simulink model "px4_rc_control"  (R2021b)
settings: Solver=FixedStepAuto  StartTime=0.0  StopTime=inf  RelTol=1e-3
undefined symbols (not defined in the file): A, B, G, R
libraries: robotlib x3, aerolibanimutils x1
settings Model: Creator=jawher  LastModifiedBy=jawher
settings OptimizationCC: EnhancedBackFolding=on  PassReuseOutputArgsAs=Individual arguments  ZeroExternalMemoryAtStartup=off  ZeroInternalMemoryAtStartup=off  MaxStackSize=64  OptimizeBlockOrder=speed  DifferentSizesBufferReuse=on  OptimizationCustomize=off  EfficientTunableParamExpr=on
settings DebuggingCC: ParameterTunabilityLossMsg=error
settings HardwareCC: ProdBitPerPointer=32  ProdBitPerSizeT=32  ProdBitPerPtrDiffT=32  ProdLargestAtomicFloat=None  ProdIntDivRoundTo=Undefined  ProdEndianess=Unspecified  ProdWordSize=32  ProdHWDeviceType=Generic->Unspecified (assume 32-bit Generic)
settings SFSimCC: MATLABDynamicMemAlloc=off
settings RTWCC: Description=Embedded Coder  SystemTargetFile=ert.tlc  HardwareBoard=Robot Operating System (ROS)  TLCOptions="-aInlineSetEventsForThisBaseRateFcn=TLC_FALSE -aSuppressMultiTaskScheduler=TLC_FALSE  -aRateBasedStepFcn=0"  TemplateMakefile=ert_default_tmf  Toolchain=Catkin  TargetLang=C++
settings CodeAppCC: ForceParamTrailComments=on  IgnoreCustomStorageClasses=off  OperatorAnnotations=on  SimulinkDataObjDesc=on  SFDataObjDesc=on  InsertBlockDesc=on

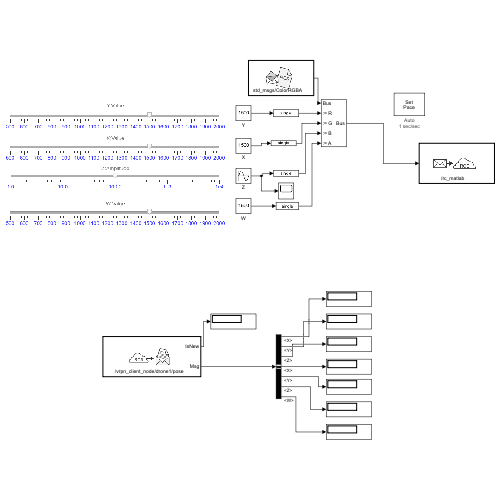
[thumbnail: Simulink's stored preview of the top-level diagram]
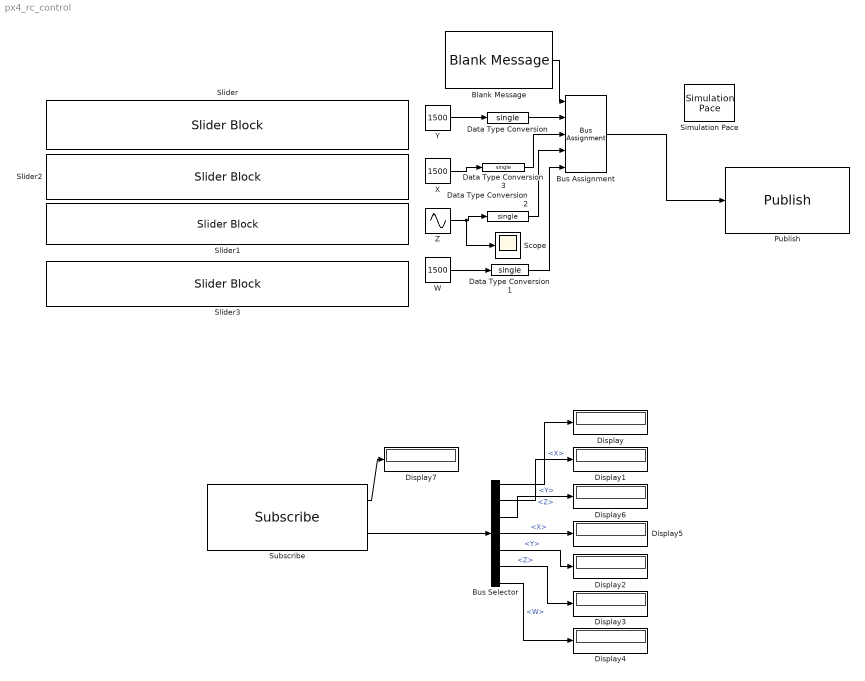
== system px4_rc_control ==
  Blank Message : robotlib/Blank Message  messageClass=Message  entityType=std_msgs/ColorRGBA  messageType=std_msgs/ColorRGBA  SampleTime=inf  legacyBusStruct=off
  Bus Assignment : BusAssignment  AssignedSignals=R,G,B,A
  Bus Selector : BusSelector  OutputSignals=Pose.Position.X,Pose.Position.Y,Pose.Position.Z,Pose.Orientation.X,Pose.Orientation.Y,Pose.Orientation.Z,Pose.Orientation.W
  Data Type Conversion{,1..3} (4 alike) : DataTypeConversion  OutDataTypeStr=single
  Display{,1..7} (8 alike) : Display
  Publish : robotlib/Publish  topicSource=Select from ROS network  topic=/rc_matlab  messageType=std_msgs/ColorRGBA  legacyBusStruct=off  messageQueueLength=10
  Scope : Scope
  Simulation Pace : aerolibanimutils/Simulation Pace  SimulationPace=1  SleepMode=Auto  OutputPaceError=off  SampleTime=1/30
  Slider : SliderBlock  ScaleMin=500  ScaleMax=2000
  Slider1 : SliderBlock  ScaleMin=1  ScaleMax=10000  ScaleType=Log
  Slider2 : SliderBlock  ScaleMin=500  ScaleMax=2000
  Slider3 : SliderBlock  ScaleMin=500  ScaleMax=2000
  Subscribe : robotlib/Subscribe  topicSource=Select from ROS network  topic=/vrpn_client_node/drone1/pose  messageType=geometry_msgs/PoseStamped  SampleTime=-1  legacyBusStruct=off  messageQueueLength=10
  W : Constant  Value=1500
  X : Constant  Value=1500
  Y : Constant  Value=1500
  Z : Sin  Amplitude=100  Bias=1200  Frequency=0.1
  wires:
  Subscribe/2 -> Bus Selector/1
  Bus Selector/1 -> Display/1  "<X>"
  Bus Selector/2 -> Display1/1  "<Y>"
  Bus Selector/7 -> Display4/1  "<W>"
  Bus Selector/6 -> Display3/1  "<Z>"
  Bus Selector/5 -> Display2/1  "<Y>"
  Bus Selector/4 -> Display5/1  "<X>"
  Bus Selector/3 -> Display6/1  "<Z>"
  Subscribe/1 -> Display7/1
  Blank Message/1 -> Bus Assignment/1
  Bus Assignment/1 -> Publish/1
  Data Type Conversion/1 -> Bus Assignment/2
  Y/1 -> Data Type Conversion/1
  Data Type Conversion3/1 -> Bus Assignment/3
  X/1 -> Data Type Conversion3/1
  Data Type Conversion2/1 -> Bus Assignment/4
  Z/1 -> Scope/1, Data Type Conversion2/1
  W/1 -> Data Type Conversion1/1
  Data Type Conversion1/1 -> Bus Assignment/5
